simulink model "ProofofScoreAlloc"  (R2023b)
settings: Solver=ode8  StartTime=0.0  StopTime=10  FixedStep=1/10  RelTol=1e-3
libraries: SignalEditorBlockLib x5
settings Model: Creator=AGBOLAND  LastModifiedBy=andrewboland
settings ModelReferenceCC: EnableRefExpFcnMdlSchedulingChecks=on

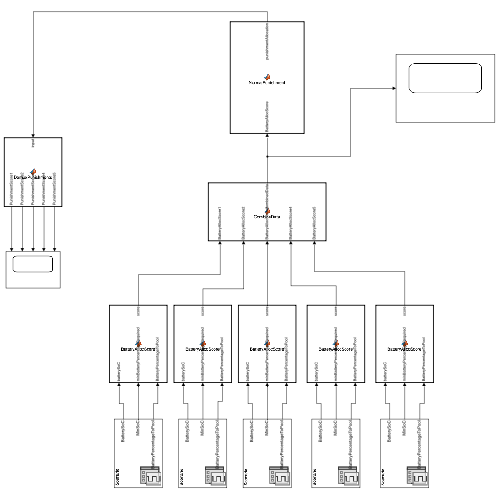
[thumbnail: Simulink's stored preview of the top-level diagram]
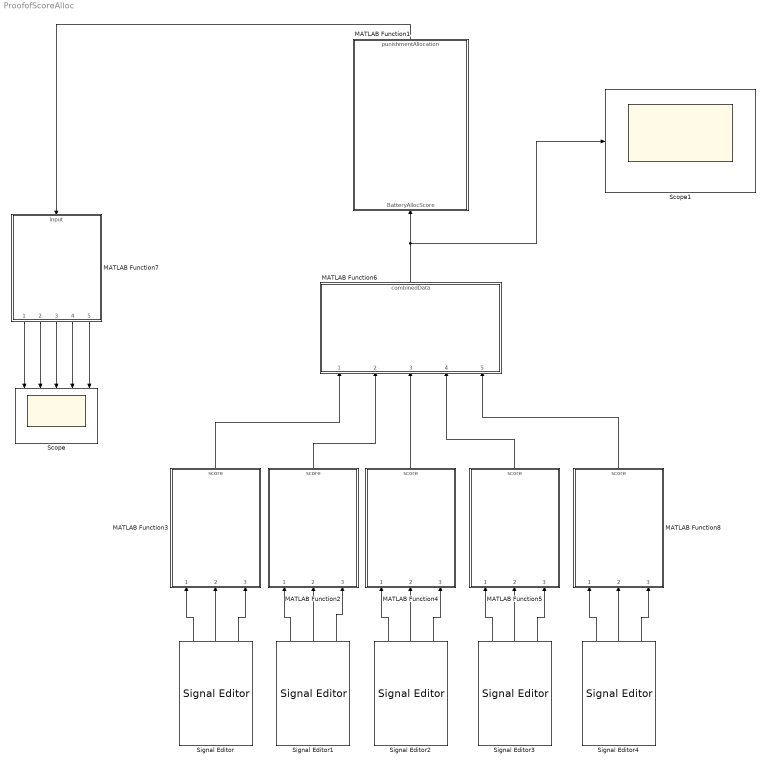
== system ProofofScoreAlloc ==
  MATLAB Function1 : MATLAB Function  TreatAsAtomicUnit=on
  MATLAB Function2 : MATLAB Function  TreatAsAtomicUnit=on
  MATLAB Function3 : MATLAB Function  TreatAsAtomicUnit=on
  MATLAB Function4 : MATLAB Function  TreatAsAtomicUnit=on
  MATLAB Function5 : MATLAB Function  TreatAsAtomicUnit=on
  MATLAB Function6 : MATLAB Function  TreatAsAtomicUnit=on
  MATLAB Function7 : MATLAB Function  TreatAsAtomicUnit=on
  MATLAB Function8 : MATLAB Function  TreatAsAtomicUnit=on
  Scope : Scope  NumInputPorts=5
  Scope1 : Scope
  Signal Editor : SignalEditorBlockLib/Signal Editor  FileName=fauxData1.mat  ActiveScenario=Scenario  ActiveSignal=BatterySoC  IsBus=off  OutputBusObjectStr=Bus: BusObject  SampleTime=0  Interpolate=off  ZeroCross=off  OutputAfterFinalValue=Setting to zero  Unit=inherit  PreserveSignalName=on  ApplySigPropsToAllScenarios=on  ApplySigPropsToAllSignals=off
  Signal Editor1 : SignalEditorBlockLib/Signal Editor  FileName=fauxData2.mat  ActiveScenario=Scenario  ActiveSignal=BatterySoC  IsBus=off  OutputBusObjectStr=Bus: BusObject  SampleTime=0  Interpolate=off  ZeroCross=off  OutputAfterFinalValue=Setting to zero  Unit=inherit  PreserveSignalName=on  ApplySigPropsToAllScenarios=on  ApplySigPropsToAllSignals=off
  Signal Editor2 : SignalEditorBlockLib/Signal Editor  FileName=fauxData3.mat  ActiveScenario=Scenario  ActiveSignal=BatterySoC  IsBus=off  OutputBusObjectStr=Bus: BusObject  SampleTime=0  Interpolate=off  ZeroCross=off  OutputAfterFinalValue=Setting to zero  Unit=inherit  PreserveSignalName=on  ApplySigPropsToAllScenarios=on  ApplySigPropsToAllSignals=off
  Signal Editor3 : SignalEditorBlockLib/Signal Editor  FileName=fauxData4.mat  ActiveScenario=Scenario  ActiveSignal=BatterySoC  IsBus=off  OutputBusObjectStr=Bus: BusObject  SampleTime=0  Interpolate=off  ZeroCross=off  OutputAfterFinalValue=Setting to zero  Unit=inherit  PreserveSignalName=on  ApplySigPropsToAllScenarios=on  ApplySigPropsToAllSignals=off
  Signal Editor4 : SignalEditorBlockLib/Signal Editor  FileName=fauxData5.mat  ActiveScenario=Scenario  ActiveSignal=BatterySoC  IsBus=off  OutputBusObjectStr=Bus: BusObject  SampleTime=0  Interpolate=off  ZeroCross=off  OutputAfterFinalValue=Setting to zero  Unit=inherit  PreserveSignalName=on  ApplySigPropsToAllScenarios=on  ApplySigPropsToAllSignals=off
  wires:
  MATLAB Function3/1(score) -> MATLAB Function6/1(BatteryAllocScore1)
  MATLAB Function2/1(score) -> MATLAB Function6/2(BatteryAllocScore2)
  MATLAB Function4/1(score) -> MATLAB Function6/3(BatteryAllocScore3)
  MATLAB Function5/1(score) -> MATLAB Function6/4(BatteryAllocScore4)
  MATLAB Function8/1(score) -> MATLAB Function6/5(BatteryAllocScore5)
  MATLAB Function6/1(combinedData) -> Scope1/1, MATLAB Function1/1(BatteryAllocScore)
  MATLAB Function7/1(PunishmentScore1) -> Scope/1
  MATLAB Function7/2(PunishmentScore2) -> Scope/2
  MATLAB Function7/3(PunishmentScore3) -> Scope/3
  MATLAB Function7/4(PunishmentScore4) -> Scope/4
  MATLAB Function7/5(PunishmentScore5) -> Scope/5
  Signal Editor/1 -> MATLAB Function3/1(batterySoC)
  Signal Editor/2 -> MATLAB Function3/2(minBatteryPercentageRequired)
  Signal Editor/3 -> MATLAB Function3/3(BatteryPercentageToPool)
  Signal Editor1/2 -> MATLAB Function2/2(minBatteryPercentageRequired)
  Signal Editor1/1 -> MATLAB Function2/1(batterySoC)
  Signal Editor1/3 -> MATLAB Function2/3(BatteryPercentageToPool)
  Signal Editor2/2 -> MATLAB Function4/2(minBatteryPercentageRequired)
  Signal Editor2/1 -> MATLAB Function4/1(batterySoC)
  Signal Editor2/3 -> MATLAB Function4/3(BatteryPercentageToPool)
  Signal Editor3/2 -> MATLAB Function5/2(minBatteryPercentageRequired)
  Signal Editor3/1 -> MATLAB Function5/1(batterySoC)
  Signal Editor3/3 -> MATLAB Function5/3(BatteryPercentageToPool)
  Signal Editor4/2 -> MATLAB Function8/2(minBatteryPercentageRequired)
  Signal Editor4/1 -> MATLAB Function8/1(batterySoC)
  Signal Editor4/3 -> MATLAB Function8/3(BatteryPercentageToPool)
  MATLAB Function1/1(punishmentAllocation) -> MATLAB Function7/1(input)

== matlab function ProofofScoreAlloc/MATLAB Function1 ==
  data: BatteryAllocScore input; punishmentAllocation output
function punishmentAllocation = NormalPunishment(BatteryAllocScore)
    % A function to find the punishment level of a load when the pool is at
    % a stable level

    % Finding the average of all BatteryAllocation Scores
    AvgBatteryAllocScore = mean(BatteryAllocScore);

    % Calculating 4 Standard Deviations away from the average
    fourStdevs = AvgBatteryAllocScore - (1.2 * std(BatteryAllocScore));

    % Calculating 2 Standard Deviations away from the average
    twoStdevs = AvgBatteryAllocScore - (1 * std(BatteryAllocScore));

    % Initialize punishmentAllocation array
    punishmentAllocation = zeros(length(BatteryAllocScore), 1);

    for i = 1:length(BatteryAllocScore)
        if BatteryAllocScore(i) < fourStdevs
            % Assigns highest punishment to loads > 4 stdevs away from mean
            punishmentAllocation(i) = 2;
        elseif BatteryAllocScore(i) < twoStdevs
            % Assigns medium punishment to loads in between 2 and 4 stdevs
            % from mean
            punishmentAllocation(i) = 1;
        else
            % Assigns no punishment to all other loads
            punishmentAllocation(i) = 0;
        end
    end
end

== matlab function ProofofScoreAlloc/MATLAB Function3 ==
  data: batterySoC input; score output; minBatteryPercentageRequired input; BatteryPercentageToPool input
function score = BatteryAllocScore(batterySoC, minBatteryPercentageRequired, ...
    BatteryPercentageToPool)
    % A function to calculate an individual load's score

    score = (BatteryPercentageToPool)...
        /(batterySoC-minBatteryPercentageRequired) * 100;
end

== matlab function ProofofScoreAlloc/MATLAB Function2 ==
  data: batterySoC input; score output; minBatteryPercentageRequired input; BatteryPercentageToPool input
function score = BatteryAllocScore(batterySoC, minBatteryPercentageRequired, ...
    BatteryPercentageToPool)
    % A function to calculate an individual load's score

    score = (BatteryPercentageToPool)...
        /(batterySoC-minBatteryPercentageRequired) * 100;
end

== matlab function ProofofScoreAlloc/MATLAB Function4 ==
  data: batterySoC input; score output; minBatteryPercentageRequired input; BatteryPercentageToPool input
function score = BatteryAllocScore(batterySoC, minBatteryPercentageRequired, ...
    BatteryPercentageToPool)
    % A function to calculate an individual load's score

    score = (BatteryPercentageToPool)...
        /(batterySoC-minBatteryPercentageRequired) * 100;
end

== matlab function ProofofScoreAlloc/MATLAB Function5 ==
  data: batterySoC input; score output; minBatteryPercentageRequired input; BatteryPercentageToPool input
function score = BatteryAllocScore(batterySoC, minBatteryPercentageRequired, ...
    BatteryPercentageToPool)
    % A function to calculate an individual load's score

    score = (BatteryPercentageToPool)...
        /(batterySoC-minBatteryPercentageRequired) * 100;
end

== matlab function ProofofScoreAlloc/MATLAB Function8 ==
  data: batterySoC input; score output; minBatteryPercentageRequired input; BatteryPercentageToPool input
function score = BatteryAllocScore(batterySoC, minBatteryPercentageRequired, ...
    BatteryPercentageToPool)
    % A function to calculate an individual load's score

    score = (BatteryPercentageToPool)...
        /(batterySoC-minBatteryPercentageRequired) * 100;
end

== matlab function ProofofScoreAlloc/MATLAB Function6 ==
  data: BatteryAllocScore1 input; combinedData output; BatteryAllocScore2 input; BatteryAllocScore3 input; BatteryAllocScore4 input; BatteryAllocScore5 input
function combinedData = CombineData(BatteryAllocScore1, BatteryAllocScore2, BatteryAllocScore3, BatteryAllocScore4, BatteryAllocScore5)

    combinedData = [BatteryAllocScore1,BatteryAllocScore2,BatteryAllocScore3,BatteryAllocScore4,BatteryAllocScore5];

end

== matlab function ProofofScoreAlloc/MATLAB Function7 ==
  data: input input; PunishmentScore1 output; PunishmentScore2 output; PunishmentScore3 output; PunishmentScore4 output; PunishmentScore5 output
function [PunishmentScore1, PunishmentScore2, PunishmentScore3, PunishmentScore4, PunishmentScore5] = DemuxPunishments(input)
    PunishmentScore1 = input(1);
    PunishmentScore2 = input(2);
    PunishmentScore3 = input(3);
    PunishmentScore4 = input(4);
    PunishmentScore5 = input(5);

end
